simulink model "current_model"  (R2019a)
settings: Solver=FixedStepAuto  StartTime=0.0  StopTime=10.0  FixedStep=0.1  RelTol=1e-3
values from neighbouring files (symbols this model uses):
  SimulationToRun = 5    [init.m]
undefined symbols (not defined in the file or in its folder): sim6CurrentAngle, useCurrentM
libraries: simulink x1
settings Model: Creator=den  LastModifiedBy=den

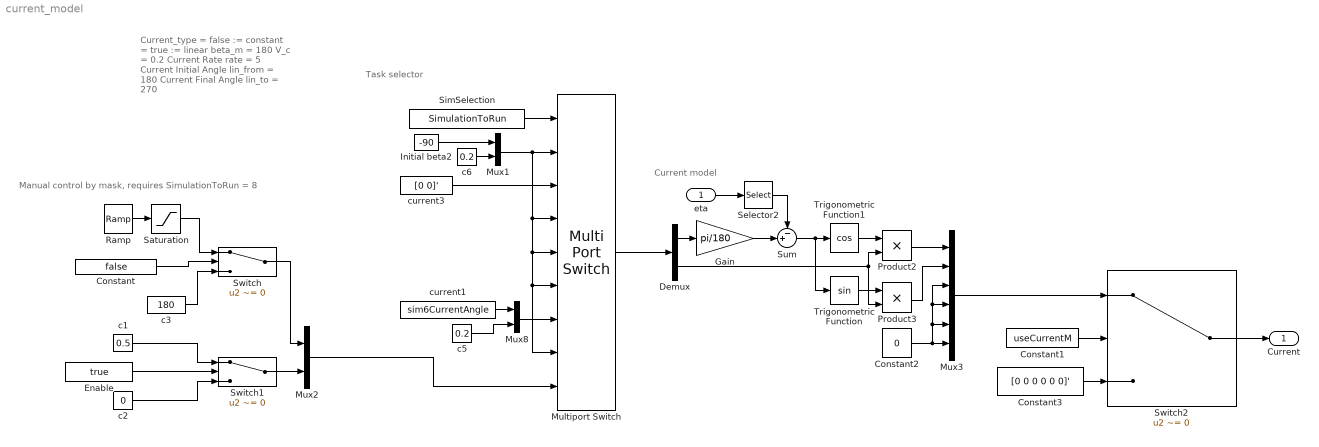
== system current_model ==
  note: Current_type = false := constant
      | 			= true := linear
      | beta_m = 180
      | V_c = 0.2
      | Current Rate
      | rate = 5
      | Current Initial Angle
      | lin_from = 180
      | Current Final Angle
      | lin_to = 270
  note: Current model
  note: Manual control by mask, requires SimulationToRun = 8
  note: Task selector
  eta : Inport  PortDimensions=3
  Constant : Constant  Value=false
  Constant1 : Constant  Value=useCurrentM
  Constant2 : Constant  Value=0
  Constant3 : Constant  Value=[0 0 0 0 0 0]'
  Demux : Demux  Outputs=2
  Enable : Constant  Value=true
  Gain : Gain  Gain=pi/180
  Initial beta2 : Constant  Value=-90
  Multiport Switch : MultiPortSwitch  Inputs=8  DiagnosticForDefault=None
  Mux1 : Mux  Inputs=2
  Mux2 : Mux  Inputs=2
  Mux3 : Mux  Inputs=6
  Mux8 : Mux  Inputs=2
  Product2 : Product
  Product3 : Product
  Ramp : simulink/Sources/Ramp  slope=1/5  start=0  InitialOutput=180
  Saturation : Saturate  UpperLimit=270  LowerLimit=180
  Selector2 : Selector  InputPortWidth=3  IndexOptions=Index vector (dialog)  Indices=3  OutputSizes=1
  SimSelection : Constant  Value=SimulationToRun
  Sum : Sum  Inputs=-+|
  Switch : Switch  Criteria=u2 ~= 0
  Switch1 : Switch  Criteria=u2 ~= 0
  Switch2 : Switch  Criteria=u2 ~= 0
  Trigonometric Function : Trigonometry
  Trigonometric Function1 : Trigonometry  Operator=cos
  c1 : Constant  Value=0.5
  c2 : Constant  Value=0
  c3 : Constant  Value=180
  c5 : Constant  Value=0.2
  c6 : Constant  Value=0.2
  current1 : Constant  Value=sim6CurrentAngle
  current3 : Constant  Value=[0 0]'
  Current : Outport  PortDimensions=6
  wires:
  Constant2/1 -> Mux3/3, Mux3/4, Mux3/5, Mux3/6
  Product3/1 -> Mux3/2
  Switch1/1 -> Mux2/2
  Demux/2 -> Product2/2, Product3/2
  Trigonometric Function1/1 -> Product2/1
  Sum/1 -> Trigonometric Function/1, Trigonometric Function1/1
  Demux/1 -> Gain/1
  c3/1 -> Switch/3
  Enable/1 -> Switch1/2
  Ramp/1 -> Saturation/1
  c6/1 -> Mux1/2
  c1/1 -> Switch1/1
  Constant/1 -> Switch/2
  Switch/1 -> Mux2/1
  Saturation/1 -> Switch/1
  Trigonometric Function/1 -> Product3/1
  SimSelection/1 -> Multiport Switch/1
  Product2/1 -> Mux3/1
  eta/1 -> Selector2/1
  c2/1 -> Switch1/3
  Selector2/1 -> Sum/1
  Gain/1 -> Sum/2
  Initial beta2/1 -> Mux1/1
  Multiport Switch/1 -> Demux/1
  current1/1 -> Mux8/1
  c5/1 -> Mux8/2
  current3/1 -> Multiport Switch/3
  Mux2/1 -> Multiport Switch/9
  Mux1/1 -> Multiport Switch/8, Multiport Switch/6, Multiport Switch/5, Multiport Switch/4, Multiport Switch/2
  Mux8/1 -> Multiport Switch/7
  Mux3/1 -> Switch2/1
  Constant3/1 -> Switch2/3
  Constant1/1 -> Switch2/2
  Switch2/1 -> Current/1
